simulink model "Demo_MinSegMega_V2"  (R2015a)
settings: Solver=FixedStepDiscrete  SolverMode=SingleTasking  StartTime=0.0  StopTime=inf  FixedStep=.03  RelTol=1e-3
libraries: MinSegLibrary_MinSegMega x4, arduinolib x4, MinSegLibrary_M2V3 x1, RASPlib x1
settings Model: SimulationMode=external  ExtModeTrigDuration=2  Creator=Alec  LastModifiedBy=hurstj
settings OptimizationCC: ExpressionDepthLimit=2147483647  OptimizeModelRefInitCode=on  LifeSpan=1
settings DebuggingCC: UnderspecifiedInitializationDetection=Classic  MergeDetectMultiDrivingBlocksExec=none  StateNameClashWarn=warning
settings HardwareCC: ProdBitPerInt=16  ProdBitPerPointer=8  ProdIntDivRoundTo=Zero  ProdEndianess=LittleEndian  ProdWordSize=8  ProdHWDeviceType=Atmel->AVR
settings RTWCC: SystemTargetFile=realtime.tlc  GenerateMakefile=off  TemplateMakefile=realtime.tmf  Description=Real-Time Toolbox  RTWVerbose=off
settings CodeAppCC: CustomSymbolStrType=$N$R$M  InternalIdentifier=Classic
settings ERTTargetCC: CombineOutputUpdateFcns=off  ExtMode=on  ExtModeTransport=3  ExtModeMexArgs=0 45 115200 30  ERTSrcFileBannerTemplate=realtime_code_template.cgt  ERTHdrFileBannerTemplate=realtime_code_template.cgt  ERTDataSrcFileTemplate=realtime_code_template.cgt  ERTDataHdrFileTemplate=realtime_code_template.cgt  ERTCustomFileTemplate=realtime_file_process.tlc

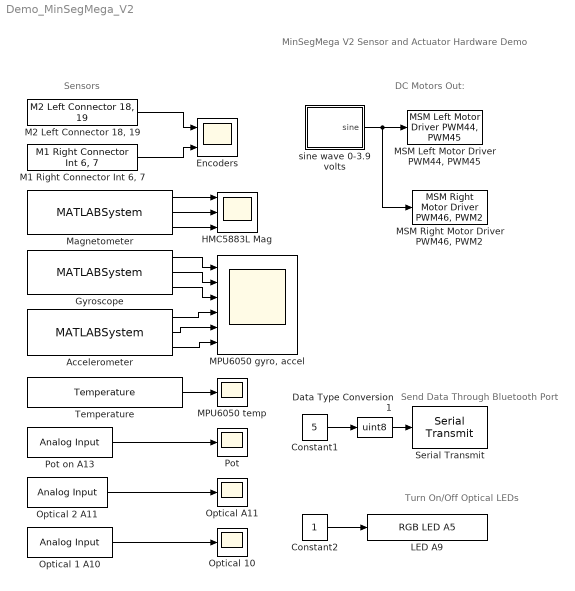
== system Demo_MinSegMega_V2 ==
  note: MinSegMega V2 Sensor and Actuator
      | Hardware Demo
  note: DC Motors Out:
  note: Sensors
  note: Send Data Through Bluetooth Port
  note: Turn On/Off Optical LEDs
  Accelerometer : MATLABSystem  System=soMPU6050Accel  SimulateUsing=Code generation
      mask Type: soMPU6050Accel
      mask Display:
      | disp('soMPU6050Accel');
      | port_label('output',1,'xaccel');
      | port_label('output',2,'yaccel');
      | port_label('output',3,'zaccel');
  Constant1 : Constant  Value=5  SampleTime=-1
  Constant2 : Constant  SampleTime=-1
  Data Type Conversion1 : DataTypeConversion  OutDataTypeStr=uint8
  Encoders : Scope  NumInputPorts=2
      settings: TimeRange=30  YMin=-203.7~-150  YMax=-184.3~400
  Gyroscope : MATLABSystem  System=soMPU6050Gyro  DLPFmode=0
      mask Type: soMPU6050Gyro
      mask Display:
      | disp('soMPU6050Gyro');
      | port_label('output',1,'xvel');
      | port_label('output',2,'yvel');
      | port_label('output',3,'zvel');
  HMC5883L Mag : Scope  NumInputPorts=3
      settings: TimeRange=10  YMin=-500~450~275  YMax=-300~775~550  SaveName=ScopeData7
  LED A9 : MinSegLibrary_M2V3/RGB LED A5  Pin=9
  "M1 Right Connector Int 6, 7" : MinSegLibrary_MinSegMega/M1 Right Connector Int 6, 7  Encoder=2  PinA=6  PinB=7
  "M2 Left Connector 18, 19" : MinSegLibrary_MinSegMega/M2 Left Connector 18, 19  Encoder=1  PinA=19  PinB=18
  "MPU6050 gyro, accel" : Scope  NumInputPorts=6
      settings: TimeRange=10  YMin=-40000~-40000~-40000~-12500~-8000~7500  YMax=40000~40000~40000~5000~3000~27500
  MPU6050 temp : Scope
      settings: TimeRange=30  YMin=-3750  YMax=-1750  SaveName=ScopeData2
  "MSM Left Motor Driver PWM44, PWM45" : MinSegLibrary_MinSegMega/MSM Left Motor Driver PWM44, PWM45  Vsupply=3.9  PWMoffset=0
  "MSM Right Motor Driver PWM46, PWM2 " : MinSegLibrary_MinSegMega/MSM Right Motor Driver PWM46, PWM2   Vsupply=3.9  PWMoffset=0
  Magnetometer : MATLABSystem  System=soHMC5883L  SimulateUsing=Code generation
      mask Type: soHMC5883L
      mask Display:
      | disp('soHMC5883L');
      | port_label('output',1,'xmag');
      | port_label('output',2,'ymag');
      | port_label('output',3,'zmag');
  "Optical 1 A10 " : arduinolib/Analog Input  pinNumber=10  sampleTime=-1  blockPlatform=arduino
  Optical 10 : Scope
      settings: TimeRange=30  YMin=300  YMax=1100  SaveName=ScopeData4
  Optical 2 A11 : arduinolib/Analog Input  pinNumber=11  sampleTime=-1  blockPlatform=arduino
  Optical A11 : Scope
      settings: TimeRange=30  YMin=100  YMax=1100  SaveName=ScopeData3
  Pot : Scope
      settings: TimeRange=30  YMin=275  YMax=600  SaveName=ScopeData6
  Pot on A13 : arduinolib/Analog Input  pinNumber=13  sampleTime=-1  blockPlatform=arduino
  Serial Transmit : arduinolib/Serial Transmit  portNumber=3  blockPlatform=arduino
  Temperature : RASPlib/Temperature  SimulateUsing=Code generation
  sine wave 0-3.9 volts : Subsystem
  wires:
  sine wave 0-3.9 volts/1(sine) -> "MSM Right Motor Driver PWM46, PWM2 "/1, "MSM Left Motor Driver PWM44, PWM45"/1
  Optical 2 A11/1 -> Optical A11/1
  Pot on A13/1 -> Pot/1
  "Optical 1 A10 "/1 -> Optical 10/1
  Magnetometer/2 -> HMC5883L Mag/2
  Magnetometer/3 -> HMC5883L Mag/3
  Magnetometer/1 -> HMC5883L Mag/1
  Gyroscope/1 -> "MPU6050 gyro, accel"/1
  Gyroscope/2 -> "MPU6050 gyro, accel"/2
  Gyroscope/3 -> "MPU6050 gyro, accel"/3
  Accelerometer/3 -> "MPU6050 gyro, accel"/6
  Accelerometer/2 -> "MPU6050 gyro, accel"/5
  Accelerometer/1 -> "MPU6050 gyro, accel"/4
  Constant1/1 -> Data Type Conversion1/1
  Data Type Conversion1/1 -> Serial Transmit/1
  "M2 Left Connector 18, 19"/1 -> Encoders/1
  "M1 Right Connector Int 6, 7"/1 -> Encoders/2
  Temperature/1 -> MPU6050 temp/1
  Constant2/1 -> LED A9/1

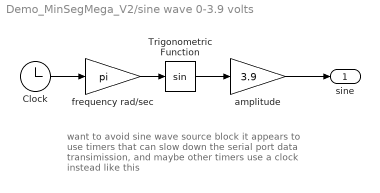
== system Demo_MinSegMega_V2/sine wave 0-3.9 volts ==
  note: want to avoid sine wave source block
      | it appears to use timers that can slow down the
      | serial port data transimission, and maybe
      | other timers
      |
      | use a clock instead like this
  Clock : Clock
  Trigonometric Function : Trigonometry
  amplitude : Gain  Gain=3.9
  frequency rad/sec : Gain  Gain=pi
  sine : Outport
  wires:
  amplitude/1 -> sine/1
  frequency rad/sec/1 -> Trigonometric Function/1
  Trigonometric Function/1 -> amplitude/1
  Clock/1 -> frequency rad/sec/1
